simulink model "model"  (R2014a)
settings: Solver=ode3  StartTime=0.0  StopTime=stop_time  FixedStep=step  RelTol=1e-3
values from neighbouring files (symbols this model uses):
  Cp = 3.2E6    (= 3200000)    [calculate.m]
  F_B = 2*0    (= 0)    [calculate.m]
  K0 = 6.5    [calculate.m]
  Kd = 80    [calculate.m]
  Kf = 10/1510    (= 0.00662251655629)    [calculate.m]
  Ku = UPm/Um    (= 30)    [calculate.m]
  Kv = 1    [calculate.m]
  Kx = 10/3.78E-5/80    (= 3306.87830688)    [calculate.m]
  m = 0.025    [calculate.m]
  Tu = 0.00005    (= 5e-05)    [calculate.m]
  U = 10    [calculate.m]
settings Model: Creator=Павел  LastModifiedBy=Павел

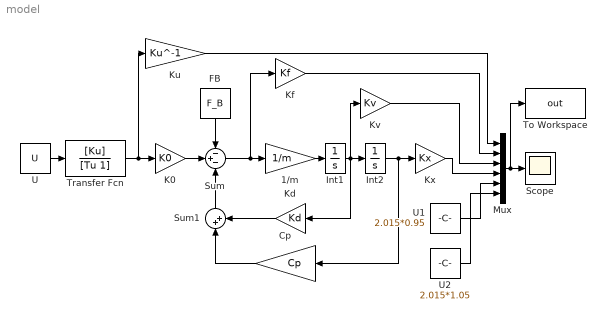
== system model ==
  1/m : Gain  Gain=1/m
  Cp : Gain  Gain=Cp
  FB : Constant  Value=F_B
  Int1 : Integrator
  Int2 : Integrator
  K0 : Gain  Gain=K0
  Kd : Gain  Gain=Kd
  Kf : Gain  Gain=Kf
  Ku : Gain  Gain=Ku^-1
  "Kv " : Gain  Gain=Kv
  "Kx " : Gain  Gain=Kx
  Mux : Mux  Inputs=6
  Scope : Scope
  Sum : Sum  Inputs=-+-
  Sum1 : Sum  Inputs=|++
  To Workspace : ToWorkspace  VariableName=out  SaveFormat=Structure With Time  SampleTime=-1
  Transfer Fcn : TransferFcn  Numerator=[Ku]  Denominator=[Tu 1]
  U : Constant  Value=U
  U1 : Constant  Value=2.015*0.95
  U2 : Constant  Value=2.015*1.05
  wires:
  Transfer Fcn/1 -> Ku/1, K0/1
  U/1 -> Transfer Fcn/1
  K0/1 -> Sum/2
  FB/1 -> Sum/1
  Sum1/1 -> Sum/3
  Kd/1 -> Sum1/2
  Cp/1 -> Sum1/1
  Sum/1 -> Kf/1, 1/m/1
  1/m/1 -> Int1/1
  Int1/1 -> "Kv "/1, Kd/1, Int2/1
  Int2/1 -> Cp/1, "Kx "/1
  "Kv "/1 -> Mux/3
  Kf/1 -> Mux/2
  Ku/1 -> Mux/1
  "Kx "/1 -> Mux/4
  Mux/1 -> To Workspace/1, Scope/1
  U1/1 -> Mux/5
  U2/1 -> Mux/6
